simulink model "RLC_Circuit_Shabbir"  (R2016a)
settings: Solver=FixedStepAuto  StartTime=0.0  StopTime=0.006  FixedStep=1e-6  RelTol=1e-3
values from neighbouring files (symbols this model uses):
  L = 1000    [simulation_2_2.m]
undefined symbols (not defined in the file or in its folder): C, R
settings Model: Creator=Iffat  LastModifiedBy=SHABBIR

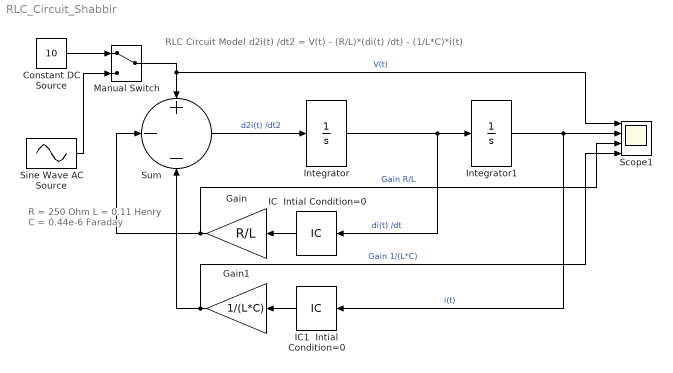
== system RLC_Circuit_Shabbir ==
  note: RLC Circuit Model d2i(t) /dt2 = V(t) - (R/L)*(di(t) /dt) - (1/L*C)*i(t)
  note: R = 250 Ohm
      | L = 0.11 Henry
      | C = 0.44e-6 Faraday
  Constant DC Source : Constant  Value=10
  Gain : Gain  Gain=R/L
  Gain1 : Gain  Gain=1/(L*C)
  IC  Intial Condition=0 : InitialCondition  Value=0
  IC1  Intial Condition=0 : InitialCondition  Value=0
  Integrator : Integrator
  Integrator1 : Integrator
  Manual Switch : ManualSwitch
  Scope1 : Scope  NumInputPorts=4
  Sine Wave AC Source : Sin  Frequency=10  SampleTime=0
  Sum : Sum  Inputs=+--
  wires:
  Sum/1 -> Integrator/1  "d2i(t) /dt2"
  Integrator/1 -> Integrator1/1, IC  Intial Condition=0/1  "di(t) /dt"
  Gain1/1 -> Scope1/4, Sum/3  "Gain 1/(L*C)"
  Integrator1/1 -> Scope1/2, IC1  Intial Condition=0/1  "i(t)"
  IC1  Intial Condition=0/1 -> Gain1/1
  IC  Intial Condition=0/1 -> Gain/1
  Constant DC Source/1 -> Manual Switch/1
  Manual Switch/1 -> Scope1/1, Sum/1  "V(t)"
  Sine Wave AC Source/1 -> Manual Switch/2
  Gain/1 -> Scope1/3, Sum/2  "Gain R/L"
